simulink model "sogi_pll"  (R2022a)
settings: Solver=FixedStepDiscrete  StartTime=0.0  StopTime=30/60  FixedStep=1/10000  MaxStep=0.0001  RelTol=1e-3
undefined symbols (not defined in the file): DiscIntNeverNeededParam
libraries: simulink_extras x1
settings Model: Creator=ra38298  LastModifiedBy=rshba
settings SolverCC: AlgebraicLoopSolver=TrustRegion
settings OptimizationCC: DefaultParameterBehavior=Inlined  UseDivisionForNetSlopeComputation=on  GainParamInheritBuiltInType=on  UseFloatMulNetSlope=on  InlineInvariantSignals=on  PassReuseOutputArgsAs=Individual arguments  ZeroExternalMemoryAtStartup=off  NoFixptDivByZeroProtection=on  EfficientFloat2IntCast=on  LifeSpan=1  OptimizationLevel=level1  OptimizationCustomize=off  EfficientTunableParamExpr=on
settings DebuggingCC: ParameterTunabilityLossMsg=error  SFUnexpectedBacktrackingDiag=warning  SFNoUnconditionalDefaultTransitionDiag=warning
settings HardwareCC: ProdBitPerChar=16  ProdBitPerInt=16  ProdBitPerPointer=32  ProdBitPerSizeT=32  ProdBitPerPtrDiffT=32  ProdLargestAtomicInteger=Integer  ProdLargestAtomicFloat=None  ProdWordSize=16  ProdLongLongMode=on  ProdHWDeviceType=Texas Instruments->C2000
settings SFSimCC: MATLABDynamicMemAlloc=off  CustomCodeUndefinedFunction=UseInterfaceOnly
settings RTWCC: SystemTargetFile=ert.tlc  GenCodeOnly=on  TemplateMakefile=ert_default_tmf  GenerateReport=on  BuildConfiguration=Debug  LaunchReport=on  DLArmComputeVersion=19.05
settings CodeAppCC: ForceParamTrailComments=on  IgnoreCustomStorageClasses=off  OperatorAnnotations=on  SimulinkDataObjDesc=on  SFDataObjDesc=on  CustomSymbolStrGlobalVar=rt$N$M  CustomSymbolStrType=$N$M  CustomSymbolStrFcn=$N$M$F  CustomSymbolStrMacro=$N$M  InsertBlockDesc=on  EnableCustomComments=on
settings ERTTargetCC: TargetLangStandard=C99 (ISO)  GenerateSampleERTMain=on  IncludeMdlTerminateFcn=off  CombineSignalStateStructs=on  SuppressErrorStatus=on  SupportAbsoluteTime=off  SupportNonFinite=off  SupportComplex=off  InlinedParameterPlacement=NonHierarchical  ERTCustomFileTemplate=example_file_process.tlc  ERTFilePackagingFormat=CompactWithDataFile

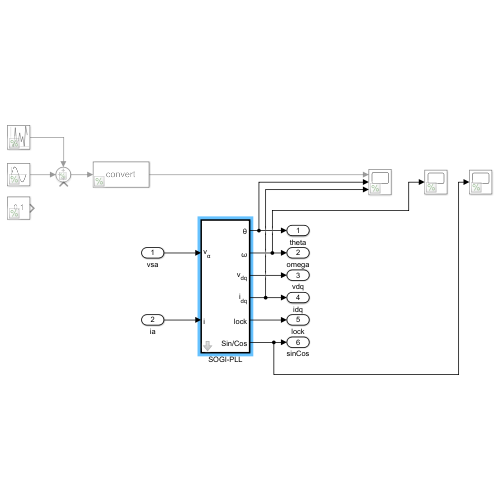
[thumbnail: Simulink's stored preview of the top-level diagram]
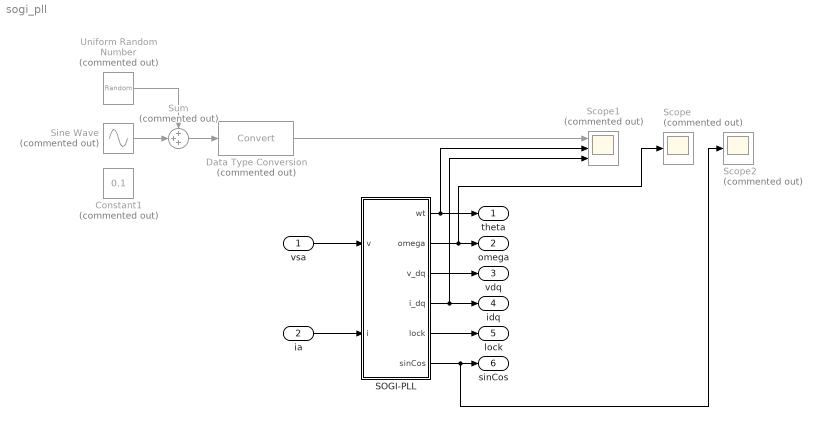
== system sogi_pll ==
  vsa : Inport
  ia : Inport  Port=2
  Constant1 : Constant  Commented=on  Value=0.1  OutDataTypeStr=single
  Data Type Conversion : DataTypeConversion  Commented=on  SaturateOnIntegerOverflow=off  RndMeth=Floor
  SOGI-PLL : Subsystem  TreatAsAtomicUnit=on  mask{fNom=60, K=0.5, B0=166.877556, B1=-166.322444}
      mask prompts: fNom "Nominal Frequency (Hz)"; K "SOGI gain (k)"; B0 "LF Coeff B0"; B1 "LF Coeff B1"
      mask DialogControl DescGroupVar Prompt: SOGI-type PLL
      mask DialogControl DescTextVar Prompt: This blocks implements a PLL based on a second order generalized integrator.
      mask Display:
      | %Print the block type:
      | color('black');
      | port_label('input',1,'v_{\alpha}','texmode','on');
      | port_label('input',2,'i','texmode','on');
      | 
      | port_label('output',1,'\theta','texmode','on');
      | port_label('output',2,'\omega','texmode','on');
      | port_label('output',3,'v_{dq}','texmode','on');
      | port_label('output',4,'i_{dq}','texmode','on');
      | port_label('output',5,'lock','texmode','on');
      | port_label('output',6,'Sin/Cos','texmode','on');
  Scope : Scope  Commented=on
  Scope1 : Scope  Commented=on  NumInputPorts=3
  Scope2 : Scope  Commented=on
  Sine Wave : Sin  Commented=on  Frequency=2*pi*60  SampleTime=0
  Sum : Sum  Commented=on  Inputs=+++
  Uniform Random Number : UniformRandomNumber  Commented=on  Minimum=-0.5  Maximum=0.5  SampleTime=0.0001
  theta : Outport
  omega : Outport  Port=2
  vdq : Outport  Port=3
  idq : Outport  Port=4
  lock : Outport  Port=5
  sinCos : Outport  Port=6
  wires:
  Sine Wave/1 -> Sum/2
  SOGI-PLL/1(wt) -> theta/1, Scope1/2
  SOGI-PLL/2(omega) -> Scope/1, omega/1
  SOGI-PLL/3(v_dq) -> vdq/1
  SOGI-PLL/4(i_dq) -> Scope1/3, idq/1
  SOGI-PLL/5(lock) -> lock/1
  Sum/1 -> Data Type Conversion/1
  SOGI-PLL/6(sinCos) -> Scope2/1, sinCos/1
  Data Type Conversion/1 -> Scope1/1
  Uniform Random Number/1 -> Sum/1
  vsa/1 -> SOGI-PLL/1(v)
  ia/1 -> SOGI-PLL/2(i)

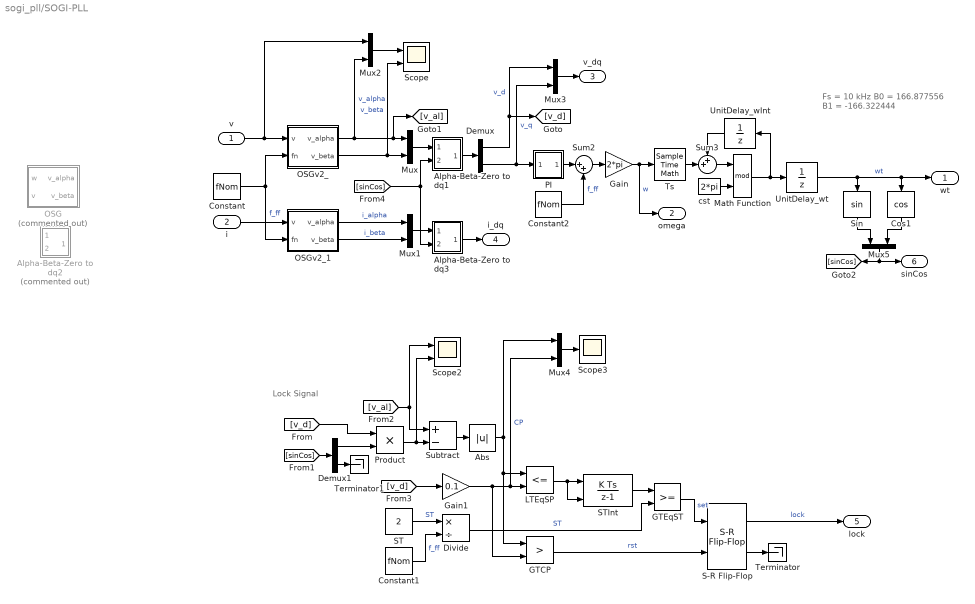
== system sogi_pll/SOGI-PLL ==
  note: Lock Signal
  note: Fs = 10 kHz
      | B0 = 166.877556
      | B1 = -166.322444
  v : Inport  OutDataTypeStr=single
  i : Inport  Port=2  OutDataTypeStr=single
  Abs : Abs  SaturateOnIntegerOverflow=off
  Alpha-Beta-Zero to dq1 : Subsystem  mask(Alpha-Beta-Zero to dq0 Transformation){KBID=kb0603}
      mask prompts: KBID "Knowledge-base id"
      mask help: Perform a transformation from a alpha-beta-zero stationary reference frame to a dq0 rotating reference frame. Angular position of the rotating frame is given by input wt (rad).
      mask Help: web(['https://imperix.ch/kb/' get_param(gcb, 'KBID') '?source=simulink&matlabversion=R' version('-release') '&libversion=' Simulink.MDLInfo('BoomBox.slx').ModelVersion])
      mask Display:
      | color('red'); plot([0 1], [0,1])
      | color('black');
      | 
      | text(0.1, 0.75, '\alpha\beta', 'horizontalAlignment','left','texmode','on');
      | text(0.95, 0.25, 'dq', 'horizontalAlignment','right');
  Alpha-Beta-Zero to dq2 : Subsystem  Commented=on  mask(Alpha-Beta-Zero to dq0 Transformation){KBID=kb0603}
      mask prompts: KBID "Knowledge-base id"
      mask help: Perform a transformation from a alpha-beta-zero stationary reference frame to a dq0 rotating reference frame. Angular position of the rotating frame is given by input wt (rad).
      mask Help: web(['https://imperix.ch/kb/' get_param(gcb, 'KBID') '?source=simulink&matlabversion=R' version('-release') '&libversion=' Simulink.MDLInfo('BoomBox.slx').ModelVersion])
      mask Display:
      | color('red'); plot([0 1], [0,1])
      | color('black');
      | 
      | text(0.1, 0.75, '\alpha\beta', 'horizontalAlignment','left','texmode','on');
      | text(0.95, 0.25, 'dq', 'horizontalAlignment','right');
  Alpha-Beta-Zero to dq3 : Subsystem  mask(Alpha-Beta-Zero to dq0 Transformation){KBID=kb0603}
      mask prompts: KBID "Knowledge-base id"
      mask help: Perform a transformation from a alpha-beta-zero stationary reference frame to a dq0 rotating reference frame. Angular position of the rotating frame is given by input wt (rad).
      mask Help: web(['https://imperix.ch/kb/' get_param(gcb, 'KBID') '?source=simulink&matlabversion=R' version('-release') '&libversion=' Simulink.MDLInfo('BoomBox.slx').ModelVersion])
      mask Display:
      | color('red'); plot([0 1], [0,1])
      | color('black');
      | 
      | text(0.1, 0.75, '\alpha\beta', 'horizontalAlignment','left','texmode','on');
      | text(0.95, 0.25, 'dq', 'horizontalAlignment','right');
  Constant : Constant  Value=fNom  OutDataTypeStr=single
  Constant1 : Constant  Value=fNom  OutDataTypeStr=single
  Constant2 : Constant  Value=fNom  OutDataTypeStr=single
  Cos1 : Trigonometry  Operator=cos
  Demux : Demux  Outputs=2
  Demux1 : Demux  Outputs=2
  Divide : Product  Inputs=*/
  GTCP : RelationalOperator  Operator=>  OutDataTypeStr=boolean  RndMeth=Simplest  InputSameDT=off
  GTEqST : RelationalOperator  OutDataTypeStr=boolean  RndMeth=Simplest  InputSameDT=off
  Gain : Gain  Gain=2*pi  OutDataTypeStr=single
  Gain1 : Gain  Gain=0.1
  LTEqSP : RelationalOperator  Operator=<=  OutDataTypeStr=boolean  RndMeth=Simplest  InputSameDT=off
  Math Function : Math  Operator=mod  SignedPower=on  OutputSignalType=real
  Mux{,1..5} (6 alike) : Mux  Inputs=2
  OSG : Subsystem  Commented=on
  OSGv2_ : Subsystem
  OSGv2_1 : Subsystem
  PI : Subsystem
  Product : Product
  S-R Flip-Flop : simulink_extras/Flip Flops/S-R Flip-Flop  initial_condition=0
  ST : Constant  Value=2
  STInt : DiscreteIntegrator  ExternalReset=falling  SampleTime=-1  OutDataTypeStr=single  LimitOutput=on  UpperSaturationLimit=single(1)  LowerSaturationLimit=single(0)  ICPrevOutput=DiscIntNeverNeededParam  ICPrevScaledInput=DiscIntNeverNeededParam
  Scope : Scope  NumInputPorts=2
  Scope2 : Scope  NumInputPorts=2
  Scope3 : Scope
  Sin : Trigonometry
  Subtract : Sum  Inputs=+-
  Sum2 : Sum  Inputs=|++
  Sum3 : Sum  Inputs=++|  OutDataTypeStr=single
  Terminator : Terminator
  Terminator1 : Terminator
  Ts : SampleTimeMath  TsampMathOp=*
  UnitDelay_wInt : UnitDelay  SampleTime=-1  HasFrameUpgradeWarning=on
  UnitDelay_wt : UnitDelay  SampleTime=-1  HasFrameUpgradeWarning=on
  cst : Constant  Value=2*pi  OutDataTypeStr=single
  wt : Outport  OutDataTypeStr=single
  omega : Outport  Port=2  OutDataTypeStr=single
  v_dq : Outport  Port=3
  i_dq : Outport  Port=4
  lock : Outport  Port=5  VectorParamsAs1DForOutWhenUnconnected=off
  sinCos : Outport  Port=6  OutDataTypeStr=single
  wires:
  PI/1(Out1) -> Sum2/1
  cst/1 -> Math Function/2
  Math Function/1 -> UnitDelay_wInt/1, UnitDelay_wt/1
  Sum3/1 -> Math Function/1
  Constant/1 -> OSGv2_1/2(fn), OSGv2_/2(fn)  "f_ff"
  OSGv2_/2(v_beta) -> Scope/2, Mux/2  "v_beta"
  UnitDelay_wt/1 -> wt/1, Cos1/1, Sin/1  "wt"
  UnitDelay_wInt/1 -> Sum3/1
  Ts/1 -> Sum3/2
  Sum2/1 -> Gain/1
  Demux/2 -> Mux3/2, PI/1(In1)  "v_q"
  Demux/1 -> Mux3/1, [v_d]  "v_d"
  OSGv2_/1(v_alpha) -> Mux/1, [v_al], Mux2/2  "v_alpha"
  Mux/1 -> Alpha-Beta-Zero to dq1/1(al_be)
  Alpha-Beta-Zero to dq1/1(dq) -> Demux/1
  [sinCos] -> Demux1/1
  [v_d] -> Product/1
  Product/1 -> Scope2/2, Subtract/2
  [v_al] -> Scope2/1, Subtract/1
  Abs/1 -> Mux4/1, LTEqSP/1, GTCP/1
  Divide/1 -> GTEqST/2  "ST"
  Gain1/1 -> GTCP/2, Mux4/2, LTEqSP/2  "CP"
  STInt/1 -> GTEqST/1
  S-R Flip-Flop/2 -> Terminator/1
  LTEqSP/1 -> STInt/1, STInt/2
  S-R Flip-Flop/1 -> lock/1  "lock"
  GTEqST/1 -> S-R Flip-Flop/1  "set"
  GTCP/1 -> S-R Flip-Flop/2  "rst"
  [v_d] -> Gain1/1
  OSGv2_1/1(v_alpha) -> Mux1/1  "i_alpha"
  OSGv2_1/2(v_beta) -> Mux1/2  "i_beta"
  v/1 -> OSGv2_/1(v), Mux2/1
  i/1 -> OSGv2_1/1(v)
  Mux2/1 -> Scope/1
  Alpha-Beta-Zero to dq3/1(dq) -> i_dq/1
  Mux3/1 -> v_dq/1
  Subtract/1 -> Abs/1
  Gain/1 -> Ts/1, omega/1  "w"
  Mux4/1 -> Scope3/1
  ST/1 -> Divide/1  "ST"
  Constant1/1 -> Divide/2  "f_ff"
  Sin/1 -> Mux5/1
  Cos1/1 -> Mux5/2
  [sinCos] -> Alpha-Beta-Zero to dq1/2(sinCos), Alpha-Beta-Zero to dq3/2(sinCos)
  Constant2/1 -> Sum2/2  "f_ff"
  Mux5/1 -> sinCos/1, [sinCos]
  Mux1/1 -> Alpha-Beta-Zero to dq3/1(al_be)
  Demux1/2 -> Terminator1/1
  Demux1/1 -> Product/2

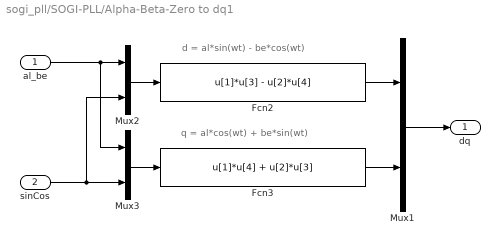
== system sogi_pll/SOGI-PLL/Alpha-Beta-Zero to dq1 ==
  note: d = al*sin(wt) - be*cos(wt)
  note: q = al*cos(wt) + be*sin(wt)
  al_be : Inport
  sinCos : Inport  Port=2
  Fcn2 : Fcn  Expr=u[1]*u[3] - u[2]*u[4]
  Fcn3 : Fcn  Expr=u[1]*u[4] + u[2]*u[3]
  Mux1 : Mux  Inputs=2
  Mux2 : Mux  Inputs=[2 2]
  Mux3 : Mux  Inputs=[2 2]
  dq : Outport
  wires:
  sinCos/1 -> Mux2/2, Mux3/2
  al_be/1 -> Mux2/1, Mux3/1
  Fcn2/1 -> Mux1/1
  Fcn3/1 -> Mux1/2
  Mux1/1 -> dq/1
  Mux3/1 -> Fcn3/1
  Mux2/1 -> Fcn2/1

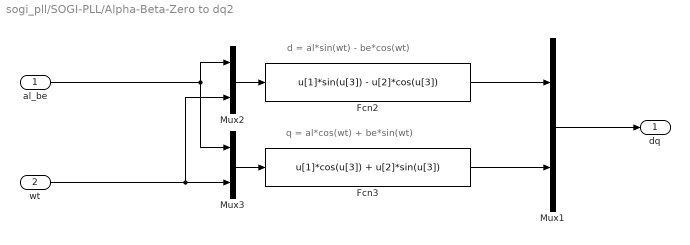
== system sogi_pll/SOGI-PLL/Alpha-Beta-Zero to dq2 ==
  note: d = al*sin(wt) - be*cos(wt)
  note: q = al*cos(wt) + be*sin(wt)
  al_be : Inport
  wt : Inport  Port=2  PortDimensions=1
  Fcn2 : Fcn  Expr=u[1]*sin(u[3]) - u[2]*cos(u[3])
  Fcn3 : Fcn  Expr=u[1]*cos(u[3]) + u[2]*sin(u[3])
  Mux1 : Mux  Inputs=2
  Mux2 : Mux  Inputs=[2 1]
  Mux3 : Mux  Inputs=[2 1]
  dq : Outport
  wires:
  wt/1 -> Mux3/2, Mux2/2
  al_be/1 -> Mux2/1, Mux3/1
  Fcn2/1 -> Mux1/1
  Fcn3/1 -> Mux1/2
  Mux1/1 -> dq/1
  Mux3/1 -> Fcn3/1
  Mux2/1 -> Fcn2/1

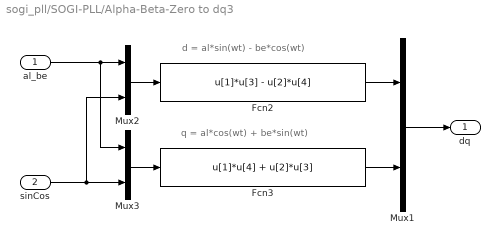
== system sogi_pll/SOGI-PLL/Alpha-Beta-Zero to dq3 ==
  note: q = al*cos(wt) + be*sin(wt)
  note: d = al*sin(wt) - be*cos(wt)
  al_be : Inport
  sinCos : Inport  Port=2
  Fcn2 : Fcn  Expr=u[1]*u[3] - u[2]*u[4]
  Fcn3 : Fcn  Expr=u[1]*u[4] + u[2]*u[3]
  Mux1 : Mux  Inputs=2
  Mux2 : Mux  Inputs=[2 2]
  Mux3 : Mux  Inputs=[2 2]
  dq : Outport
  wires:
  Mux2/1 -> Fcn2/1
  Mux3/1 -> Fcn3/1
  Mux1/1 -> dq/1
  Fcn3/1 -> Mux1/2
  Fcn2/1 -> Mux1/1
  al_be/1 -> Mux3/1, Mux2/1
  sinCos/1 -> Mux3/2, Mux2/2

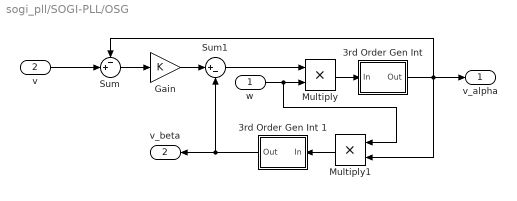
== system sogi_pll/SOGI-PLL/OSG ==
  w : Inport  OutDataTypeStr=single
  v : Inport  Port=2  OutDataTypeStr=single
  3rd Order Gen Int : Subsystem
  3rd Order Gen Int 1 : Subsystem
  Gain : Gain  Gain=K  OutDataTypeStr=single
  Multiply : Product
  Multiply1 : Product
  Sum : Sum  Inputs=-+|
  Sum1 : Sum  Inputs=|+-
  v_alpha : Outport
  v_beta : Outport  Port=2  OutDataTypeStr=single
  wires:
  w/1 -> Multiply1/1, Multiply/2
  Sum/1 -> Gain/1
  Gain/1 -> Sum1/1
  v/1 -> Sum/2
  Multiply1/1 -> 3rd Order Gen Int 1/1(In)
  Sum1/1 -> Multiply/1
  3rd Order Gen Int/1(Out) -> v_alpha/1, Multiply1/2, Sum/1
  3rd Order Gen Int 1/1(Out) -> v_beta/1, Sum1/2
  Multiply/1 -> 3rd Order Gen Int/1(In)

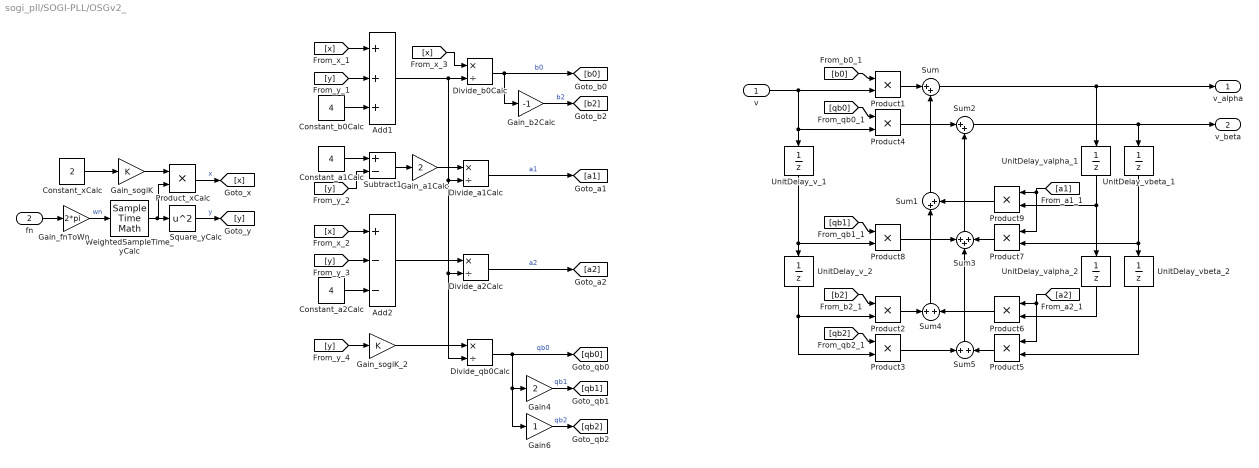
== system sogi_pll/SOGI-PLL/OSGv2_ ==
  v : Inport  OutDataTypeStr=single
  fn : Inport  Port=2  OutDataTypeStr=single
  Add1 : Sum  Inputs=+++
  Add2 : Sum  Inputs=+--
  Constant_a1Calc : Constant  Value=4  OutDataTypeStr=single
  Constant_a2Calc : Constant  Value=4  OutDataTypeStr=single
  Constant_b0Calc : Constant  Value=4  OutDataTypeStr=single
  Constant_xCalc : Constant  Value=2  OutDataTypeStr=single
  Divide_a1Calc : Product  Inputs=*/
  Divide_a2Calc : Product  Inputs=*/
  Divide_b0Calc : Product  Inputs=*/
  Divide_qb0Calc : Product  Inputs=*/
  Gain4 : Gain  Gain=2
  Gain6 : Gain
  Gain_a1Calc : Gain  Gain=2
  Gain_b2Calc : Gain  Gain=-1
  Gain_fnToWn : Gain  Gain=2*pi  OutDataTypeStr=single
  Gain_sogiK : Gain  Gain=K  OutDataTypeStr=single
  Gain_sogiK_2 : Gain  Gain=K  OutDataTypeStr=single
  Product{1..9} (9 alike) : Product
  Product_xCalc : Product
  Square_yCalc : Math  Operator=square
  Subtract1 : Sum  Inputs=+-
  Sum : Sum  Inputs=|++
  Sum1 : Sum  Inputs=|++
  Sum2 : Sum  Inputs=|++
  Sum3 : Sum  Inputs=+++
  Sum4 : Sum  Inputs=+|+
  Sum5 : Sum  Inputs=+|+
  UnitDelay_v_1 : UnitDelay  SampleTime=-1  HasFrameUpgradeWarning=on
  UnitDelay_v_2 : UnitDelay  SampleTime=-1  HasFrameUpgradeWarning=on
  UnitDelay_valpha_1 : UnitDelay  SampleTime=-1  HasFrameUpgradeWarning=on
  UnitDelay_valpha_2 : UnitDelay  SampleTime=-1  HasFrameUpgradeWarning=on
  UnitDelay_vbeta_1 : UnitDelay  SampleTime=-1  HasFrameUpgradeWarning=on
  UnitDelay_vbeta_2 : UnitDelay  SampleTime=-1  HasFrameUpgradeWarning=on
  WeightedSampleTime_yCalc : SampleTimeMath  TsampMathOp=*
  v_alpha : Outport
  v_beta : Outport  Port=2  OutDataTypeStr=single
  wires:
  Constant_xCalc/1 -> Gain_sogiK/1
  Gain_sogiK/1 -> Product_xCalc/1
  WeightedSampleTime_yCalc/1 -> Product_xCalc/2, Square_yCalc/1
  Divide_b0Calc/1 -> [b0], Gain_b2Calc/1  "b0"
  Subtract1/1 -> Gain_a1Calc/1
  Gain_b2Calc/1 -> [b2]  "b2"
  Gain_sogiK_2/1 -> Divide_qb0Calc/1
  Divide_qb0Calc/1 -> [qb0], Gain4/1, Gain6/1  "qb0"
  Gain4/1 -> [qb1]  "qb1"
  fn/1 -> Gain_fnToWn/1
  Product_xCalc/1 -> [x]  "x"
  Square_yCalc/1 -> [y]  "y"
  [x] -> Add1/1
  [y] -> Add1/2
  Constant_b0Calc/1 -> Add1/3
  Add1/1 -> Divide_a2Calc/2, Divide_qb0Calc/2, Divide_a1Calc/2, Divide_b0Calc/2
  [x] -> Divide_b0Calc/1
  Constant_a1Calc/1 -> Subtract1/1
  [y] -> Subtract1/2
  Gain_a1Calc/1 -> Divide_a1Calc/1
  Constant_a2Calc/1 -> Add2/3
  [y] -> Add2/2
  [x] -> Add2/1
  Add2/1 -> Divide_a2Calc/1
  [y] -> Gain_sogiK_2/1
  Divide_a1Calc/1 -> [a1]  "a1"
  Divide_a2Calc/1 -> [a2]  "a2"
  Gain6/1 -> [qb2]  "qb2"
  Sum2/1 -> v_beta/1, UnitDelay_vbeta_1/1
  Product1/1 -> Sum/1
  UnitDelay_v_1/1 -> Product8/2, UnitDelay_v_2/1
  UnitDelay_vbeta_1/1 -> UnitDelay_vbeta_2/1, Product7/2
  UnitDelay_valpha_1/1 -> Product9/2, UnitDelay_valpha_2/1
  Sum/1 -> v_alpha/1, UnitDelay_valpha_1/1
  [b0] -> Product1/1
  [b2] -> Product2/1
  UnitDelay_v_2/1 -> Product3/2, Product2/2
  [qb2] -> Product3/1
  [qb0] -> Product4/1
  Product4/1 -> Sum2/1
  v/1 -> Product1/2, UnitDelay_v_1/1, Product4/2
  Product2/1 -> Sum4/1
  Sum1/1 -> Sum/2
  Product8/1 -> Sum3/1
  Sum3/1 -> Sum2/2
  Product3/1 -> Sum5/1
  Sum4/1 -> Sum1/1
  Sum5/1 -> Sum3/2
  Product5/1 -> Sum5/2
  Product6/1 -> Sum4/2
  UnitDelay_valpha_2/1 -> Product6/2
  UnitDelay_vbeta_2/1 -> Product5/2
  [a2] -> Product5/1, Product6/1
  [a1] -> Product7/1, Product9/1
  Product7/1 -> Sum3/3
  Product9/1 -> Sum1/2
  Gain_fnToWn/1 -> WeightedSampleTime_yCalc/1  "wn"
  [qb1] -> Product8/1

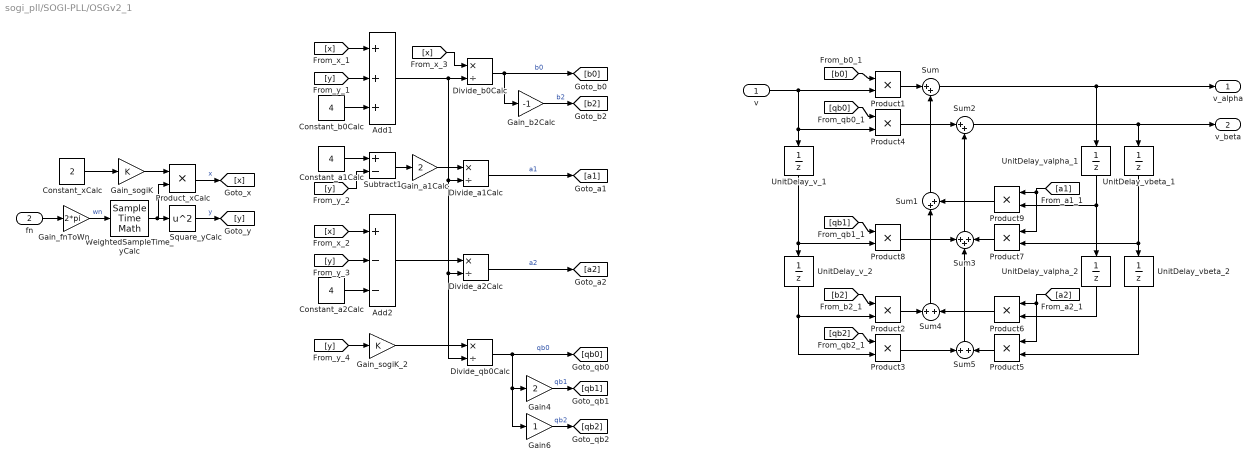
== system sogi_pll/SOGI-PLL/OSGv2_1 ==
  v : Inport  OutDataTypeStr=single
  fn : Inport  Port=2  OutDataTypeStr=single
  Add1 : Sum  Inputs=+++
  Add2 : Sum  Inputs=+--
  Constant_a1Calc : Constant  Value=4  OutDataTypeStr=single
  Constant_a2Calc : Constant  Value=4  OutDataTypeStr=single
  Constant_b0Calc : Constant  Value=4  OutDataTypeStr=single
  Constant_xCalc : Constant  Value=2  OutDataTypeStr=single
  Divide_a1Calc : Product  Inputs=*/
  Divide_a2Calc : Product  Inputs=*/
  Divide_b0Calc : Product  Inputs=*/
  Divide_qb0Calc : Product  Inputs=*/
  Gain4 : Gain  Gain=2
  Gain6 : Gain
  Gain_a1Calc : Gain  Gain=2
  Gain_b2Calc : Gain  Gain=-1
  Gain_fnToWn : Gain  Gain=2*pi  OutDataTypeStr=single
  Gain_sogiK : Gain  Gain=K  OutDataTypeStr=single
  Gain_sogiK_2 : Gain  Gain=K  OutDataTypeStr=single
  Product{1..9} (9 alike) : Product
  Product_xCalc : Product
  Square_yCalc : Math  Operator=square
  Subtract1 : Sum  Inputs=+-
  Sum : Sum  Inputs=|++
  Sum1 : Sum  Inputs=|++
  Sum2 : Sum  Inputs=|++
  Sum3 : Sum  Inputs=+++
  Sum4 : Sum  Inputs=+|+
  Sum5 : Sum  Inputs=+|+
  UnitDelay_v_1 : UnitDelay  SampleTime=-1  HasFrameUpgradeWarning=on
  UnitDelay_v_2 : UnitDelay  SampleTime=-1  HasFrameUpgradeWarning=on
  UnitDelay_valpha_1 : UnitDelay  SampleTime=-1  HasFrameUpgradeWarning=on
  UnitDelay_valpha_2 : UnitDelay  SampleTime=-1  HasFrameUpgradeWarning=on
  UnitDelay_vbeta_1 : UnitDelay  SampleTime=-1  HasFrameUpgradeWarning=on
  UnitDelay_vbeta_2 : UnitDelay  SampleTime=-1  HasFrameUpgradeWarning=on
  WeightedSampleTime_yCalc : SampleTimeMath  TsampMathOp=*
  v_alpha : Outport
  v_beta : Outport  Port=2  OutDataTypeStr=single
  wires:
  [qb1] -> Product8/1
  Gain_fnToWn/1 -> WeightedSampleTime_yCalc/1  "wn"
  Product9/1 -> Sum1/2
  Product7/1 -> Sum3/3
  [a1] -> Product9/1, Product7/1
  [a2] -> Product6/1, Product5/1
  UnitDelay_vbeta_2/1 -> Product5/2
  UnitDelay_valpha_2/1 -> Product6/2
  Product6/1 -> Sum4/2
  Product5/1 -> Sum5/2
  Sum5/1 -> Sum3/2
  Sum4/1 -> Sum1/1
  Product3/1 -> Sum5/1
  Sum3/1 -> Sum2/2
  Product8/1 -> Sum3/1
  Sum1/1 -> Sum/2
  Product2/1 -> Sum4/1
  v/1 -> Product4/2, UnitDelay_v_1/1, Product1/2
  Product4/1 -> Sum2/1
  [qb0] -> Product4/1
  [qb2] -> Product3/1
  UnitDelay_v_2/1 -> Product2/2, Product3/2
  [b2] -> Product2/1
  [b0] -> Product1/1
  Sum/1 -> UnitDelay_valpha_1/1, v_alpha/1
  UnitDelay_valpha_1/1 -> UnitDelay_valpha_2/1, Product9/2
  UnitDelay_vbeta_1/1 -> Product7/2, UnitDelay_vbeta_2/1
  UnitDelay_v_1/1 -> UnitDelay_v_2/1, Product8/2
  Product1/1 -> Sum/1
  Sum2/1 -> UnitDelay_vbeta_1/1, v_beta/1
  Gain6/1 -> [qb2]  "qb2"
  Divide_a2Calc/1 -> [a2]  "a2"
  Divide_a1Calc/1 -> [a1]  "a1"
  [y] -> Gain_sogiK_2/1
  Add2/1 -> Divide_a2Calc/1
  [x] -> Add2/1
  [y] -> Add2/2
  Constant_a2Calc/1 -> Add2/3
  Gain_a1Calc/1 -> Divide_a1Calc/1
  [y] -> Subtract1/2
  Constant_a1Calc/1 -> Subtract1/1
  [x] -> Divide_b0Calc/1
  Add1/1 -> Divide_b0Calc/2, Divide_a1Calc/2, Divide_qb0Calc/2, Divide_a2Calc/2
  Constant_b0Calc/1 -> Add1/3
  [y] -> Add1/2
  [x] -> Add1/1
  Square_yCalc/1 -> [y]  "y"
  Product_xCalc/1 -> [x]  "x"
  fn/1 -> Gain_fnToWn/1
  Gain4/1 -> [qb1]  "qb1"
  Divide_qb0Calc/1 -> Gain6/1, Gain4/1, [qb0]  "qb0"
  Gain_sogiK_2/1 -> Divide_qb0Calc/1
  Gain_b2Calc/1 -> [b2]  "b2"
  Subtract1/1 -> Gain_a1Calc/1
  Divide_b0Calc/1 -> Gain_b2Calc/1, [b0]  "b0"
  WeightedSampleTime_yCalc/1 -> Square_yCalc/1, Product_xCalc/2
  Gain_sogiK/1 -> Product_xCalc/1
  Constant_xCalc/1 -> Gain_sogiK/1

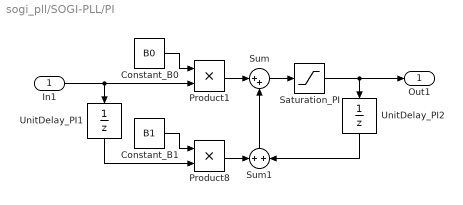
== system sogi_pll/SOGI-PLL/PI ==
  In1 : Inport
  Constant_B0 : Constant  Value=B0
  Constant_B1 : Constant  Value=B1
  Product1 : Product
  Product8 : Product
  Saturation_PI : Saturate  UpperLimit=20  LowerLimit=-20
  Sum : Sum  Inputs=|++
  Sum1 : Sum  Inputs=+|+
  UnitDelay_PI1 : UnitDelay  SampleTime=-1  HasFrameUpgradeWarning=on
  UnitDelay_PI2 : UnitDelay  SampleTime=-1  HasFrameUpgradeWarning=on
  Out1 : Outport
  wires:
  Sum1/1 -> Sum/2
  Sum/1 -> Saturation_PI/1
  Product1/1 -> Sum/1
  Constant_B0/1 -> Product1/1
  Product8/1 -> Sum1/1
  In1/1 -> UnitDelay_PI1/1, Product1/2
  UnitDelay_PI2/1 -> Sum1/2
  UnitDelay_PI1/1 -> Product8/2
  Constant_B1/1 -> Product8/1
  Saturation_PI/1 -> Out1/1, UnitDelay_PI2/1

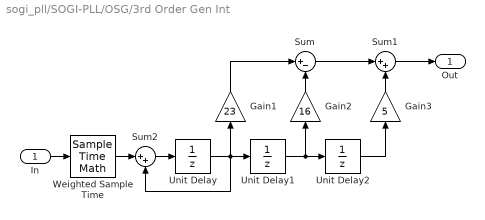
== system sogi_pll/SOGI-PLL/OSG/3rd Order Gen Int ==
  In : Inport  OutDataTypeStr=single
  Gain1 : Gain  Gain=23  OutDataTypeStr=single
  Gain2 : Gain  Gain=16  OutDataTypeStr=single
  Gain3 : Gain  Gain=5  OutDataTypeStr=single
  Sum : Sum  Inputs=|+-
  Sum1 : Sum  Inputs=|++
  Sum2 : Sum  Inputs=|++
  Unit Delay : UnitDelay  SampleTime=-1  HasFrameUpgradeWarning=on
  Unit Delay1 : UnitDelay  SampleTime=-1  HasFrameUpgradeWarning=on
  Unit Delay2 : UnitDelay  SampleTime=-1  HasFrameUpgradeWarning=on
  Weighted Sample Time : SampleTimeMath  TsampMathOp=*  weightValue=1.0/12.0
  Out : Outport
  wires:
  Sum2/1 -> Unit Delay/1
  Weighted Sample Time/1 -> Sum2/1
  Sum1/1 -> Out/1
  Sum/1 -> Sum1/1
  Gain3/1 -> Sum1/2
  Gain1/1 -> Sum/1
  Gain2/1 -> Sum/2
  Unit Delay2/1 -> Gain3/1
  Unit Delay/1 -> Gain1/1, Sum2/2, Unit Delay1/1
  Unit Delay1/1 -> Gain2/1, Unit Delay2/1
  In/1 -> Weighted Sample Time/1

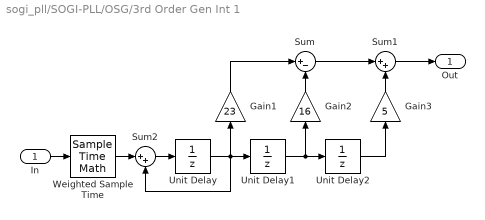
== system sogi_pll/SOGI-PLL/OSG/3rd Order Gen Int 1 ==
  In : Inport  OutDataTypeStr=single
  Gain1 : Gain  Gain=23  OutDataTypeStr=single
  Gain2 : Gain  Gain=16  OutDataTypeStr=single
  Gain3 : Gain  Gain=5  OutDataTypeStr=single
  Sum : Sum  Inputs=|+-
  Sum1 : Sum  Inputs=|++
  Sum2 : Sum  Inputs=|++
  Unit Delay : UnitDelay  SampleTime=-1  HasFrameUpgradeWarning=on
  Unit Delay1 : UnitDelay  SampleTime=-1  HasFrameUpgradeWarning=on
  Unit Delay2 : UnitDelay  SampleTime=-1  HasFrameUpgradeWarning=on
  Weighted Sample Time : SampleTimeMath  TsampMathOp=*  weightValue=1.0/12.0
  Out : Outport
  wires:
  In/1 -> Weighted Sample Time/1
  Unit Delay1/1 -> Unit Delay2/1, Gain2/1
  Unit Delay/1 -> Unit Delay1/1, Sum2/2, Gain1/1
  Unit Delay2/1 -> Gain3/1
  Gain2/1 -> Sum/2
  Gain1/1 -> Sum/1
  Gain3/1 -> Sum1/2
  Sum/1 -> Sum1/1
  Sum1/1 -> Out/1
  Weighted Sample Time/1 -> Sum2/1
  Sum2/1 -> Unit Delay/1
